simulink model "GlbDa_LSum"  (R2016b)
settings: configuration reference "CodeGenConfigSet" (kept outside this file)
values from neighbouring files (symbols this model uses):
  GlbDa_LSum_lVehCHGECU_C = Calibration.Parameter    [init_GlbDa_LSum.m]
  GlbDa_LSum_VehThreshold_C = Calibration.Parameter    [init_GlbDa_LSum.m]
undefined symbols (not defined in the file or in its folder): GlbDa_LSum_DT
settings Model: Creator=zhoutinglin  LastModifiedBy=wangrui
settings ConfigSetRef: SourceLocation=Base Workspace

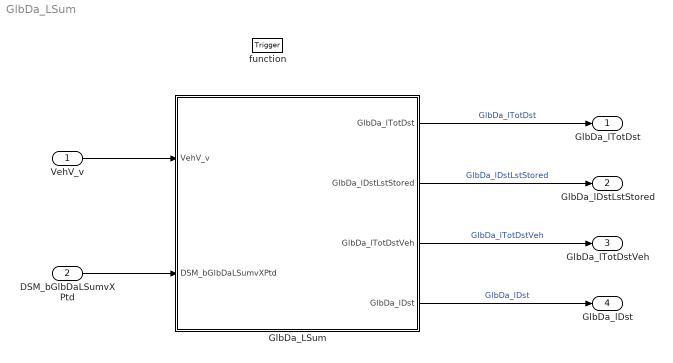
== system GlbDa_LSum ==
  VehV_v : Inport  Tag=km/h  Description=Vehicle speed  OutMin=0  OutMax=250  OutDataTypeStr=VehSpeed_km_h
  DSM_bGlbDaLSumvXPtd : Inport  Description=Enable condition for reading velocity  Port=2  OutMin=0  OutMax=1  OutDataTypeStr=boolean
  function : TriggerPort  TriggerType=function-call  VariantControl=Variant
  GlbDa_LSum : Subsystem
  GlbDa_lTotDst : Outport  Tag=Km  Description=total distance since first start  OutMin=0  OutMax=2147483  OutDataTypeStr=Length_Km
  GlbDa_lDstLstStored : Outport  Tag=Km  Description=last value of total distance in EEP  Port=2  OutMin=0  OutMax=2147483  OutDataTypeStr=Length_Km
  GlbDa_lTotDstVeh : Outport  Tag=Km  Description=total travelled distance of vehicle  Port=3  OutMin=0  OutMax=2147483  OutDataTypeStr=Length_Km
  GlbDa_lDst : Outport  Tag=m  Description=travelled distance in this drive cycle  Port=4  OutMin=0  OutMax=2147483  OutDataTypeStr=Length_m
  wires:
  VehV_v/1 -> GlbDa_LSum/1(VehV_v)
  DSM_bGlbDaLSumvXPtd/1 -> GlbDa_LSum/2(DSM_bGlbDaLSumvXPtd)
  GlbDa_LSum/1(GlbDa_lTotDst) -> GlbDa_lTotDst/1  "GlbDa_lTotDst"
  GlbDa_LSum/2(GlbDa_lDstLstStored) -> GlbDa_lDstLstStored/1  "GlbDa_lDstLstStored"
  GlbDa_LSum/3(GlbDa_lTotDstVeh) -> GlbDa_lTotDstVeh/1  "GlbDa_lTotDstVeh"
  GlbDa_LSum/4(GlbDa_lDst) -> GlbDa_lDst/1  "GlbDa_lDst"

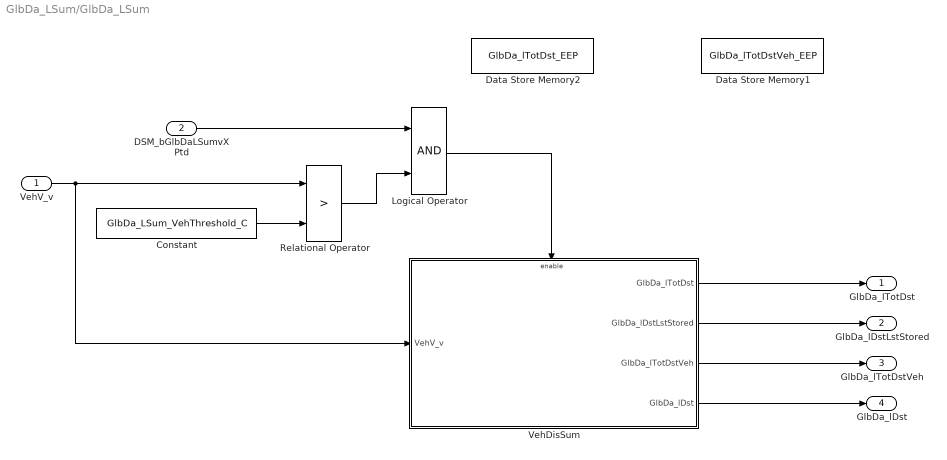
== system GlbDa_LSum/GlbDa_LSum ==
  VehV_v : Inport
  DSM_bGlbDaLSumvXPtd : Inport  Port=2
  Constant : Constant  Value=GlbDa_LSum_VehThreshold_C
  Data Store Memory1 : DataStoreMemory  DataStoreName=GlbDa_lTotDstVeh_EEP  ReadBeforeWriteMsg=warning  WriteAfterWriteMsg=warning  WriteAfterReadMsg=warning  ShowAdditionalParam=off  OutDataTypeStr=fixdt(1,32,1/1000,0)
  Data Store Memory2 : DataStoreMemory  DataStoreName=GlbDa_lTotDst_EEP  ReadBeforeWriteMsg=warning  WriteAfterWriteMsg=warning  WriteAfterReadMsg=warning  ShowAdditionalParam=off  OutDataTypeStr=fixdt(1,32,1/1000,0)
  Logical Operator : Logic  AllPortsSameDT=off  OutDataTypeStr=boolean
  Relational Operator : RelationalOperator  Operator=>  OutDataTypeStr=boolean  RndMeth=Simplest  InputSameDT=on
  VehDisSum : Subsystem  TreatAsAtomicUnit=on
  GlbDa_lTotDst : Outport
  GlbDa_lDstLstStored : Outport  Port=2
  GlbDa_lTotDstVeh : Outport  Port=3
  GlbDa_lDst : Outport  Port=4
  wires:
  VehV_v/1 -> VehDisSum/1(VehV_v), Relational Operator/1
  Constant/1 -> Relational Operator/2
  Relational Operator/1 -> Logical Operator/2
  DSM_bGlbDaLSumvXPtd/1 -> Logical Operator/1
  Logical Operator/1 -> VehDisSum/Enable
  VehDisSum/1(GlbDa_lTotDst) -> GlbDa_lTotDst/1
  VehDisSum/2(GlbDa_lDstLstStored) -> GlbDa_lDstLstStored/1
  VehDisSum/3(GlbDa_lTotDstVeh) -> GlbDa_lTotDstVeh/1
  VehDisSum/4(GlbDa_lDst) -> GlbDa_lDst/1

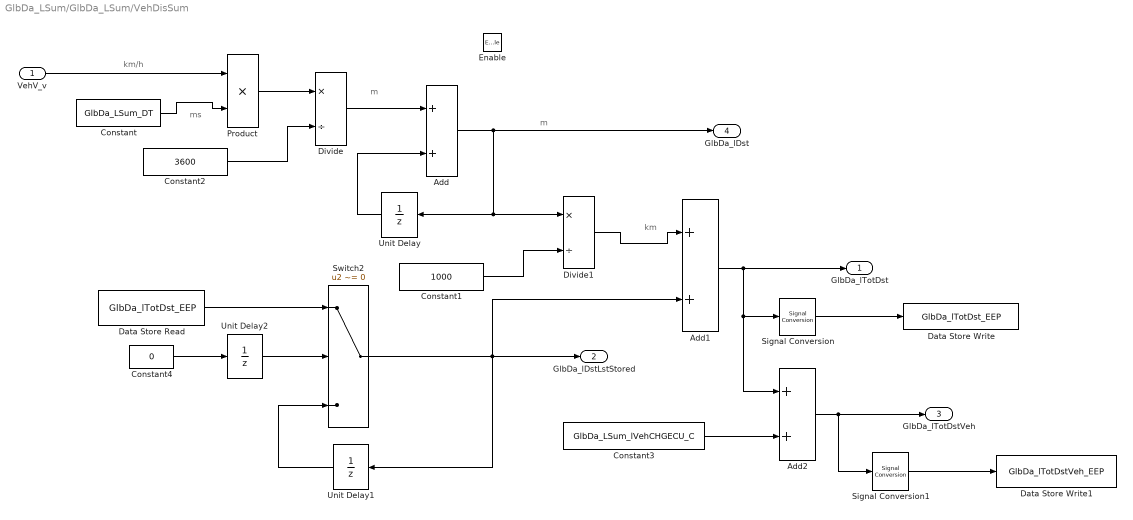
== system GlbDa_LSum/GlbDa_LSum/VehDisSum ==
  note: km
  note: m
  note: m
  note: km/h
  note: ms
  VehV_v : Inport
  Enable : EnablePort
  Add : Sum
  Add1 : Sum  OutDataTypeStr=Inherit: Inherit via back propagation  InputSameDT=on
  Add2 : Sum
  Constant : Constant  Value=GlbDa_LSum_DT
  Constant1 : Constant  Value=1000  OutDataTypeStr=uint16
  Constant2 : Constant  Value=3600  OutDataTypeStr=uint16
  Constant3 : Constant  Value=GlbDa_LSum_lVehCHGECU_C
  Constant4 : Constant  Value=0  OutDataTypeStr=boolean
  Data Store Read : DataStoreRead  DataStoreName=GlbDa_lTotDst_EEP
  Data Store Write : DataStoreWrite  DataStoreName=GlbDa_lTotDst_EEP
  Data Store Write1 : DataStoreWrite  DataStoreName=GlbDa_lTotDstVeh_EEP
  Divide : Product  Inputs=*/  OutDataTypeStr=fixdt(1,32,0.001,0)
  Divide1 : Product  Inputs=*/  OutDataTypeStr=Inherit: Inherit via back propagation
  Product : Product  OutDataTypeStr=fixdt(1,32,0.001,0)
  Signal Conversion : SignalConversion  OverrideOpt=off
  Signal Conversion1 : SignalConversion  OverrideOpt=off
  Switch2 : Switch  Criteria=u2 ~= 0  SaturateOnIntegerOverflow=on  InputSameDT=on
  Unit Delay : UnitDelay  SampleTime=-1
      settings: AttributesFormatString=InitialValue=%<InitialCondition>
  Unit Delay1 : UnitDelay  SampleTime=-1
      settings: AttributesFormatString=InitialValue=%<InitialCondition>
  Unit Delay2 : UnitDelay  InitialCondition=true  SampleTime=-1
      settings: AttributesFormatString=InitialValue=%<InitialCondition>
  GlbDa_lTotDst : Outport
  GlbDa_lDstLstStored : Outport  Port=2
  GlbDa_lTotDstVeh : Outport  Port=3
  GlbDa_lDst : Outport  Port=4
  wires:
  VehV_v/1 -> Product/1
  Constant2/1 -> Divide/2
  Constant/1 -> Product/2
  Product/1 -> Divide/1
  Divide/1 -> Add/1
  Add/1 -> Unit Delay/1, Divide1/1, GlbDa_lDst/1
  Unit Delay/1 -> Add/2
  Constant1/1 -> Divide1/2
  Divide1/1 -> Add1/1
  Constant3/1 -> Add2/2
  Switch2/1 -> Add1/2, GlbDa_lDstLstStored/1, Unit Delay1/1
  Constant4/1 -> Unit Delay2/1
  Unit Delay2/1 -> Switch2/2
  Unit Delay1/1 -> Switch2/3
  Add1/1 -> Signal Conversion/1, Add2/1, GlbDa_lTotDst/1
  Add2/1 -> Signal Conversion1/1, GlbDa_lTotDstVeh/1
  Signal Conversion/1 -> Data Store Write/1
  Signal Conversion1/1 -> Data Store Write1/1
  Data Store Read/1 -> Switch2/1
